simulink model "model"  (R2015a)
settings: Solver=ode45  StartTime=0.0  StopTime=10.0  RelTol=1e-3
values from neighbouring files (symbols this model uses):
  sampling_time = 0.02    [run_simulation.m]
undefined symbols (not defined in the file or in its folder): Ke, Kp, MIO, National_Instruments, PCI
libraries: sldrtlib x3
settings Model: Creator=Alunos  LastModifiedBy=Alunos

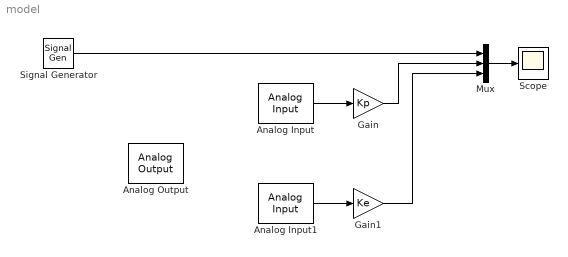
== system model ==
  Analog Input : sldrtlib/Analog Input  SampleTime=sampling_time  MaxMissedTicks=10  ShowMissedTicks=off  YieldWhenWaiting=off  DrvName=National_Instruments/PCI-MIO-16E-4  DrvAddress=4294967295  DrvOptions=[0 0 0 0 0 0]  Channels=1  RangeMode=1  VoltRange=1  DataType=1
      settings: AttributesFormatString=National Instruments\nPCI-MIO-16E-4 [auto]
  Analog Input1 : sldrtlib/Analog Input  SampleTime=sampling_time  MaxMissedTicks=10  ShowMissedTicks=off  YieldWhenWaiting=off  DrvName=National_Instruments/PCI-MIO-16E-4  DrvAddress=4294967295  DrvOptions=[0 0 0 0 0 0]  Channels=2  RangeMode=1  VoltRange=1  DataType=1
      settings: AttributesFormatString=National Instruments\nPCI-MIO-16E-4 [auto]
  Analog Output : sldrtlib/Analog Output  SampleTime=sampling_time  MaxMissedTicks=10  ShowMissedTicks=off  YieldWhenWaiting=off  DrvName=National_Instruments/PCI-MIO-16E-4  DrvAddress=4294967295  DrvOptions=[0 0 0 0 0 0]  Channels=1  RangeMode=1  VoltRange=1  InitialValue=0  FinalValue=0
      settings: AttributesFormatString=National Instruments\nPCI-MIO-16E-4 [auto]
  Gain : Gain  Gain=Kp
  Gain1 : Gain  Gain=Ke
  Mux : Mux  Inputs=3
  Scope : Scope
      settings: SaveName=scopeData  SampleInput=on  SampleTime=sampling_time
  Signal Generator : SignalGenerator  WaveForm=square  Frequency=0.4
  wires:
  Signal Generator/1 -> Mux/1
  Analog Input/1 -> Gain/1
  Analog Input1/1 -> Gain1/1
  Mux/1 -> Scope/1
  Gain/1 -> Mux/2
  Gain1/1 -> Mux/3
